simulink model "soc_dvbs2_hwtop"  (R2025b)
settings: Solver=VariableStepAuto  StartTime=0.0  StopTime=0.25  RelTol=1e-3  EnableMultiTasking=on
PreLoadFcn:
  | addpath(fullfile(matlabroot,'toolbox','whdl','whdlexamples','whdlexamples'));
InitFcn:
  | addpath(fullfile(matlabroot,'toolbox','whdl','whdlexamples','whdlexamples'));
  | soc_dvbs2_init;
values from neighbouring files (symbols this model uses):
  fs = Rsym *32    (= 128000000)    [soc_dvbs2_init.m]
  Rsym = 4e6    (= 4000000)    [soc_dvbs2_init.m]
undefined symbols (not defined in the file or in its folder): Fs, I, Q
libraries: hwlogicconnlib x2, hdlsllib x2, xilinxrfsoclib x1
CloseFcn:
  | h = warning('off','MATLAB:rmpath:DirNotFound');
  | rmpath(fullfile(matlabroot,'toolbox','whdl','whdlexamples','whdlexamples'));
  | warning(h);clear h;
settings Model: SimulationMode=accelerator  Creator=The MathWorks, Inc.  LastModifiedBy=The MathWorks, Inc.
settings SolverCC: PositivePriorityOrder=on
settings OptimizationCC: DefaultParameterBehavior=Inlined  EnhancedBackFolding=on  PassReuseOutputArgsAs=Individual arguments  ZeroExternalMemoryAtStartup=off  ZeroInternalMemoryAtStartup=off  MaxStackSize=64  OptimizeBlockOrder=speed  DifferentSizesBufferReuse=on  OptimizationCustomize=off  EfficientTunableParamExpr=on
settings DebuggingCC: ParameterTunabilityLossMsg=error
settings HardwareCC: ProdBitPerLong=64.0  ProdLargestAtomicInteger=LongLong  ProdLargestAtomicFloat=Double  ProdLongLongMode=on  ProdHWDeviceType=ARM Compatible->ARM Cortex-A (64-bit)  HardwareBoardFeatureSet=SoCBlockset
settings ModelReferenceCC: ModelReferenceNumInstancesAllowed=Single
settings SFSimCC: MATLABDynamicMemAlloc=off
settings RTWCC: SystemTargetFile=ert.tlc  HardwareBoard=Xilinx Zynq UltraScale+ RFSoC ZCU111 Evaluation Kit  TLCOptions="-aInlineSetEventsForThisBaseRateFcn=TLC_FALSE -aSuppressMultiTaskScheduler=TLC_FALSE  -aRateBasedStepFcn=0"  TemplateMakefile=ert_default_tmf  Toolchain=Linaro AArch64 Linux v6.3.1  Description=Embedded Coder
settings CodeAppCC: ForceParamTrailComments=on  IgnoreCustomStorageClasses=off  OperatorAnnotations=on  SimulinkDataObjDesc=on  SFDataObjDesc=on  InsertBlockDesc=on

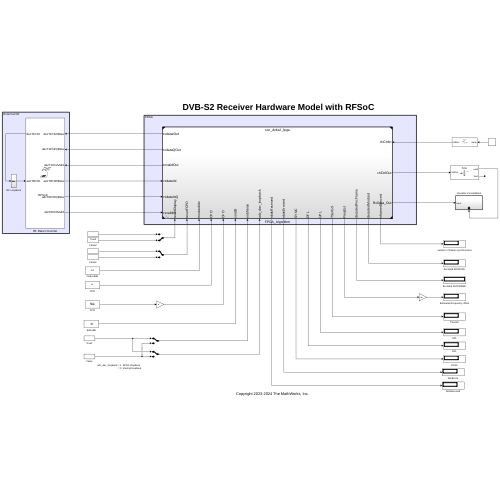
[thumbnail: Simulink's stored preview of the top-level diagram]
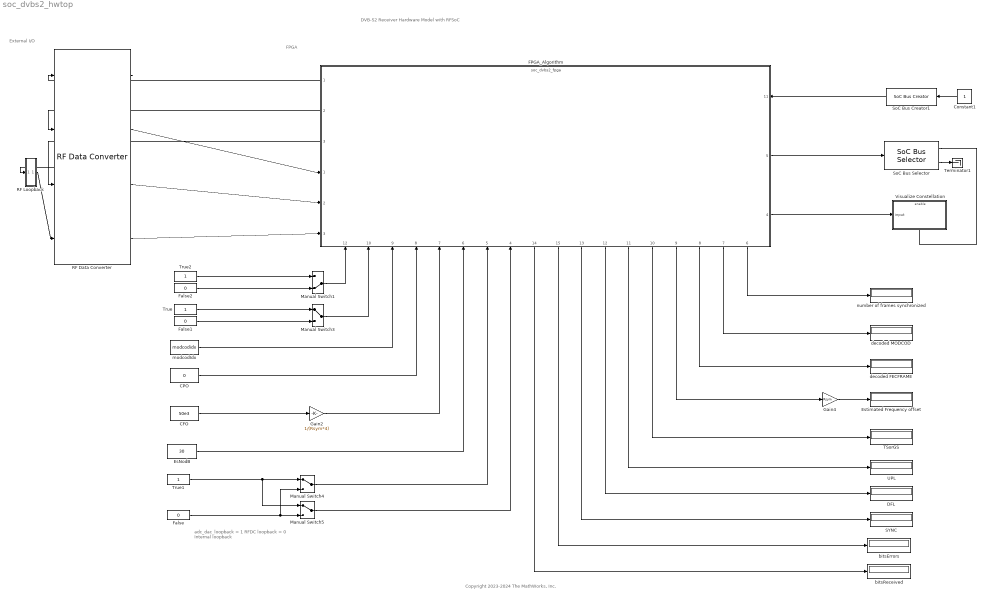
== system soc_dvbs2_hwtop ==
  note: DVB-S2 Receiver Hardware Model with RFSoC
  note: adc_dac_loopback = 1  RFDC loopback
      |                                = 0  Internal loopback
  note: External I/O
  note: FPGA
  note: Copyright 2023-2024 The MathWorks, Inc.
  CFO : Constant  Value=50e3  SampleTime=1/fs
  CPO : Constant  Value=0  OutDataTypeStr=Inherit: Inherit via back propagation  SampleTime=1/fs
  Constant1 : Constant  OutDataTypeStr=boolean  SampleTime=-1
  DFL : Display
      settings: Format=hex (Stored Integer)
  EsNodB : Constant  Value=30  OutDataTypeStr=Inherit: Inherit via back propagation  SampleTime=1/fs
  Estimated Frequency offset : Display
  FPGA_Algorithm : ModelReference  ModelNameDialog=soc_dvbs2_fpga.slx  ModelReferenceVersion=9.0
      settings: PortSchema="{\"entries\":[{\"content\":{\"sides\":[{\"content\":{\"connectorIds\":[\"Out1\",\"Out2\",\"Out3\",\"In1\",\"In2\",\"In3\"]},\"type\":\"ConnectorPlacement.EquallySpacedRectSide\",\"uuid\":\"5a98e095-40d9-43f8-91e5-a805a03516fd\"},{\"content\":{\"connectorIds\":[\"In11\",\"Out5\",\"Out4\"],\"side\":\"RIGHT\"},\"type\":\"ConnectorPlacement.EquallySpacedRectSide\",\"uuid\":\"242f1ec7-c947-482c-82ab-d4fa225331bb\"},{\"content\":{\"side\":\"TOP\"},\"type\":\"ConnectorPlacement.EquallySpacedRectSide\",\"uuid\":\"d3f55be4-91f3-4b02-af75-0bf7e7e1b925\"},{\"content\":{\"connectorIds\":[\"In12\",\"In10\",\"In9\",\"In8\",\"In7\",\"In6\",\"In5\",\"In4\",\"Out14\",\"Out15\",\"Out13\",\"Out12\",\"Out11\",\"Out10\",\"Out9\",\"Out8\",\"Out7\",\"Out6\"],\"side\":\"BOTTOM\"},\"type\":\"ConnectorPlacement.EquallySpacedRectSide\",\"uuid\":\"11ee90da-1deb-4c1f-bd41-f9aa9c63736b\"}]},\"type\":\"ConnectorPlacement.EquallySpacedConnector\",\"uuid\":\"1ac0077b-1539-4750-8893-00c30e797fc3\"}],\"packageUris\":[\"http://schema.mathworks.com/mf0/Connector/R2020b\"],\"version\":\"1.0\"}"
  False : Constant  Value=0  OutDataTypeStr=boolean  SampleTime=1/fs
  False1 : Constant  Value=0  OutDataTypeStr=boolean  SampleTime=1/fs
  False2 : Constant  Value=0  OutDataTypeStr=boolean  SampleTime=1/fs
  Gain2 : Gain  Gain=1/(Rsym*4)  OutDataTypeStr=fixdt(1,21,21)
  Gain4 : Gain  Gain=Rsym  ParamDataTypeStr=double
  Manual Switch1 : ManualSwitch  CurrentSetting=0
  Manual Switch3 : ManualSwitch
  Manual Switch4 : ManualSwitch
  Manual Switch5 : ManualSwitch
  RF Data Converter : xilinxrfsoclib/RF Data Converter  RFDCSim=Pass-through  tabPromptsCB=0  RFInterface=Customize  digitalInterface=I/Q  dac11Enable=off  dac12Enable=off  dac13Enable=off  dac14Enable=off  dac21Enable=off  dac22Enable=off  dac23Enable=on  dac24Enable=off  dac31Enable=off  dac32Enable=off  dac33Enable=off  dac34Enable=off  dac41Enable=off  dac42Enable=off  dac43Enable=off  dac44Enable=off  matchDACParam=on  dacSampleRate=2048  dacDatapathMode=Full Nyquist (0 to Fs/2)  interpolationMode=4  dacSamplesPerCycle=4  dacMixerType=Fine  dacMixerMode=I/Q->Real  dacMixerFrequency=Fs/2  dacNCOFrequency=[0.860]  dacNCOPhase=[0]  invertSyncFilter=off  dacTile1SampleRate=1000  dac11DatapathMode=Full Nyquist (0 to Fs/2)  dac11InterpolationMode=2  dac11SamplesPerCycle=2  dac11MixerType=Coarse  dac11MixerMode=I/Q->Real  dac11MixerFrequency=Fs/2  dac11NCOFrequency=0  dac11NCOPhase=0  dac11InvertSyncFilter=off  dac12DatapathMode=Full Nyquist (0 to Fs/2)  dac12InterpolationMode=2  dac12SamplesPerCycle=2  dac12MixerType=Coarse  dac12MixerMode=I/Q->Real  dac12MixerFrequency=Fs/2  dac12NCOFrequency=0  dac12NCOPhase=0  dac12InvertSyncFilter=off  dac13DatapathMode=Full Nyquist (0 to Fs/2)  dac13InterpolationMode=2  dac13SamplesPerCycle=2  dac13MixerType=Coarse  dac13MixerMode=I/Q->Real  dac13MixerFrequency=Fs/2  dac13NCOFrequency=0  dac13NCOPhase=0  dac13InvertSyncFilter=off  dac14DatapathMode=Full Nyquist (0 to Fs/2)  dac14InterpolationMode=2  dac14SamplesPerCycle=2  dac14MixerType=Coarse  dac14MixerMode=I/Q->Real  dac14MixerFrequency=Fs/2  dac14NCOFrequency=0  dac14NCOPhase=0  dac14InvertSyncFilter=off  dacTile2SampleRate=1000  dac21DatapathMode=Full Nyquist (0 to Fs/2)  dac21InterpolationMode=2  dac21SamplesPerCycle=2  dac21MixerType=Coarse  dac21MixerMode=I/Q->Real  dac21MixerFrequency=Fs/2  dac21NCOFrequency=0  dac21NCOPhase=0  dac21InvertSyncFilter=off  dac22DatapathMode=Full Nyquist (0 to Fs/2)  dac22InterpolationMode=2  dac22SamplesPerCycle=2  dac22MixerType=Coarse  dac22MixerMode=I/Q->Real  dac22MixerFrequency=Fs/2  dac22NCOFrequency=0  dac22NCOPhase=0  dac22InvertSyncFilter=off  dac23DatapathMode=Full Nyquist (0 to Fs/2)  dac23InterpolationMode=2  dac23SamplesPerCycle=2  dac23MixerType=Coarse  dac23MixerMode=I/Q->Real  dac23MixerFrequency=Fs/2  dac23NCOFrequency=0  dac23NCOPhase=0  dac23InvertSyncFilter=off  dac24DatapathMode=Full Nyquist (0 to Fs/2)  dac24InterpolationMode=2  dac24SamplesPerCycle=2  dac24MixerType=Coarse  dac24MixerMode=I/Q->Real  dac24MixerFrequency=Fs/2  dac24NCOFrequency=0  dac24NCOPhase=0  dac24InvertSyncFilter=off  dacTile3SampleRate=1000  dac31DatapathMode=Full Nyquist (0 to Fs/2)  dac31InterpolationMode=2  dac31SamplesPerCycle=2  dac31MixerType=Coarse  dac31MixerMode=I/Q->Real  dac31MixerFrequency=Fs/2  dac31NCOFrequency=0  dac31NCOPhase=0  dac31InvertSyncFilter=off  dac32DatapathMode=Full Nyquist (0 to Fs/2)  dac32InterpolationMode=2  dac32SamplesPerCycle=2  dac32MixerType=Coarse  dac32MixerMode=I/Q->Real  dac32MixerFrequency=Fs/2  dac32NCOFrequency=0  dac32NCOPhase=0  dac32InvertSyncFilter=off  dac33DatapathMode=Full Nyquist (0 to Fs/2)  dac33InterpolationMode=2  dac33SamplesPerCycle=2  dac33MixerType=Coarse  dac33MixerMode=I/Q->Real  dac33MixerFrequency=Fs/2  dac33NCOFrequency=0  dac33NCOPhase=0  dac33InvertSyncFilter=off  dac34DatapathMode=Full Nyquist (0 to Fs/2)  dac34InterpolationMode=2  dac34SamplesPerCycle=2  dac34MixerType=Coarse  dac34MixerMode=I/Q->Real  dac34MixerFrequency=Fs/2  dac34NCOFrequency=0  dac34NCOPhase=0  dac34InvertSyncFilter=off  dacTile4SampleRate=1000  dac41DatapathMode=Full Nyquist (0 to Fs/2)  dac41InterpolationMode=2  dac41SamplesPerCycle=2  dac41MixerType=Coarse  dac41MixerMode=I/Q->Real  dac41MixerFrequency=Fs/2  dac41NCOFrequency=0  dac41NCOPhase=0  dac41InvertSyncFilter=off  dac42DatapathMode=Full Nyquist (0 to Fs/2)  dac42InterpolationMode=2  dac42SamplesPerCycle=2  dac42MixerType=Coarse  dac42MixerMode=I/Q->Real  dac42MixerFrequency=Fs/2  dac42NCOFrequency=0  dac42NCOPhase=0  dac42InvertSyncFilter=off  dac43DatapathMode=Full Nyquist (0 to Fs/2)  dac43InterpolationMode=2  dac43SamplesPerCycle=2  dac43MixerType=Coarse  dac43MixerMode=I/Q->Real  dac43MixerFrequency=Fs/2  dac43NCOFrequency=0  dac43NCOPhase=0  dac43InvertSyncFilter=off  dac44DatapathMode=Full Nyquist (0 to Fs/2)  dac44InterpolationMode=2  dac44SamplesPerCycle=2  dac44MixerType=Coarse  dac44MixerMode=I/Q->Real  dac44MixerFrequency=Fs/2  dac44NCOFrequency=0  dac44NCOPhase=0  dac44InvertSyncFilter=off  adc11Enable=on  adc12Enable=off  adc13Enable=off  adc14Enable=off  adc21Enable=off  adc22Enable=off  adc23Enable=off  adc24Enable=off  adc31Enable=off  adc32Enable=off  adc33Enable=off  adc34Enable=off  adc41Enable=off  adc42Enable=off  adc43Enable=off  adc44Enable=off  adcOutUnpackedData=on  matchADCParam=on  adcSampleRate=2048  decimationMode=4  adcSamplesPerCycle=4  adcMixerType=Fine  adcMixerMode=Real->I/Q  adcMixerFrequency=Fs/2  adcNCOFrequency=[-0.860]  adcNCOPhase=[0]  adcTile1SampleRate=1000  adc11DecimationMode=2  adc11SamplesPerCycle=2  adc11MixerType=Coarse  adc11MixerMode=Real->I/Q  adc11MixerFrequency=Fs/2  adc11NCOFrequency=0  adc11NCOPhase=0  adc12DecimationMode=2  adc12SamplesPerCycle=2  adc12MixerType=Coarse  adc12MixerMode=Real->I/Q  adc12MixerFrequency=Fs/2  adc12NCOFrequency=0  adc12NCOPhase=0  adc13DecimationMode=2  adc13SamplesPerCycle=2  adc13MixerType=Coarse  adc13MixerMode=Real->I/Q  adc13MixerFrequency=Fs/2  adc13NCOFrequency=0  adc13NCOPhase=0  adc14DecimationMode=2  adc14SamplesPerCycle=2  adc14MixerType=Coarse  adc14MixerMode=Real->I/Q  adc14MixerFrequency=Fs/2  adc14NCOFrequency=0  adc14NCOPhase=0  adcTile2SampleRate=1000  adc21DecimationMode=2  adc21SamplesPerCycle=2  adc21MixerType=Coarse  adc21MixerMode=Real->I/Q  adc21MixerFrequency=Fs/2  adc21NCOFrequency=0  adc21NCOPhase=0  adc22DecimationMode=2  adc22SamplesPerCycle=2  adc22MixerType=Coarse  adc22MixerMode=Real->I/Q  adc22MixerFrequency=Fs/2  adc22NCOFrequency=0  adc22NCOPhase=0  adc23DecimationMode=2  adc23SamplesPerCycle=2  adc23MixerType=Coarse  adc23MixerMode=Real->I/Q  adc23MixerFrequency=Fs/2  adc23NCOFrequency=0  adc23NCOPhase=0  adc24DecimationMode=2  adc24SamplesPerCycle=2  adc24MixerType=Coarse  adc24MixerMode=Real->I/Q  adc24MixerFrequency=Fs/2  adc24NCOFrequency=0  adc24NCOPhase=0  adcTile3SampleRate=1000  adc31DecimationMode=2  adc31SamplesPerCycle=2  adc31MixerType=Coarse  adc31MixerMode=Real->I/Q  adc31MixerFrequency=Fs/2  adc31NCOFrequency=0  adc31NCOPhase=0  adc32DecimationMode=2  adc32SamplesPerCycle=2  adc32MixerType=Coarse  adc32MixerMode=Real->I/Q  adc32MixerFrequency=Fs/2  adc32NCOFrequency=0  adc32NCOPhase=0  adc33DecimationMode=2  adc33SamplesPerCycle=2  adc33MixerType=Coarse  adc33MixerMode=Real->I/Q  adc33MixerFrequency=Fs/2  adc33NCOFrequency=0  adc33NCOPhase=0  adc34DecimationMode=2  adc34SamplesPerCycle=2  adc34MixerType=Coarse  adc34MixerMode=Real->I/Q  adc34MixerFrequency=Fs/2  adc34NCOFrequency=0  adc34NCOPhase=0  adcTile4SampleRate=1000  adc41DecimationMode=2  adc41SamplesPerCycle=2  adc41MixerType=Coarse  adc41MixerMode=Real->I/Q  adc41MixerFrequency=Fs/2  adc41NCOFrequency=0  adc41NCOPhase=0  adc42DecimationMode=2  adc42SamplesPerCycle=2  adc42MixerType=Coarse  adc42MixerMode=Real->I/Q  adc42MixerFrequency=Fs/2  adc42NCOFrequency=0  adc42NCOPhase=0  adc43DecimationMode=2  adc43SamplesPerCycle=2  adc43MixerType=Coarse  adc43MixerMode=Real->I/Q  adc43MixerFrequency=Fs/2  adc43NCOFrequency=0  adc43NCOPhase=0  adc44DecimationMode=2  adc44SamplesPerCycle=2  adc44MixerType=Coarse  adc44MixerMode=Real->I/Q  adc44MixerFrequency=Fs/2  adc44NCOFrequency=0  adc44NCOPhase=0  multiTileSync=off  externalPLL=off  dacRealTimeNCOPortsEnable=off  adcRealTimeNCOPortsEnable=off  adcRealTimePortsEnable=off  adcThresholdMode=Sticky over  adcThreshold1=0  adcDelayCounter=0  adcThreshold2Mode=Sticky over  adcThreshold2=0  adcThreshold2DelayCounter=0  adc11ThresholdMode=Sticky over  adc11Threshold1=0  adc11DelayCounter=0  adc11Threshold2Mode=Sticky over  adc11Threshold2=0  adc11Threshold2DelayCounter=0  adc12ThresholdMode=Sticky over  adc12Threshold1=0  adc12DelayCounter=0  adc12Threshold2Mode=Sticky over  adc12Threshold2=0  adc12Threshold2DelayCounter=0  adc13ThresholdMode=Sticky over  adc13Threshold1=0  adc13DelayCounter=0  adc13Threshold2Mode=Sticky over  adc13Threshold2=0  adc13Threshold2DelayCounter=0  adc14ThresholdMode=Sticky over  adc14Threshold1=0  adc14DelayCounter=0  adc14Threshold2Mode=Sticky over  adc14Threshold2=0  adc14Threshold2DelayCounter=0  adc21ThresholdMode=Sticky over  adc21Threshold1=0  adc21DelayCounter=0  adc21Threshold2Mode=Sticky over  adc21Threshold2=0  adc21Threshold2DelayCounter=0  adc22ThresholdMode=Sticky over  adc22Threshold1=0  adc22DelayCounter=0  adc22Threshold2Mode=Sticky over  adc22Threshold2=0  adc22Threshold2DelayCounter=0  adc23ThresholdMode=Sticky over  adc23Threshold1=0  adc23DelayCounter=0  adc23Threshold2Mode=Sticky over  adc23Threshold2=0  adc23Threshold2DelayCounter=0  adc24ThresholdMode=Sticky over  adc24Threshold1=0  adc24DelayCounter=0  adc24Threshold2Mode=Sticky over  adc24Threshold2=0  adc24Threshold2DelayCounter=0  adc31ThresholdMode=Sticky over  adc31Threshold1=0  adc31DelayCounter=0  adc31Threshold2Mode=Sticky over  adc31Threshold2=0  adc31Threshold2DelayCounter=0  adc32ThresholdMode=Sticky over  adc32Threshold1=0  adc32DelayCounter=0  adc32Threshold2Mode=Sticky over  adc32Threshold2=0  adc32Threshold2DelayCounter=0  adc33ThresholdMode=Sticky over  adc33Threshold1=0  adc33DelayCounter=0  adc33Threshold2Mode=Sticky over  adc33Threshold2=0  adc33Threshold2DelayCounter=0  adc34ThresholdMode=Sticky over  adc34Threshold1=0  adc34DelayCounter=0  adc34Threshold2Mode=Sticky over  adc34Threshold2=0  adc34Threshold2DelayCounter=0  adc41ThresholdMode=Sticky over  adc41Threshold1=0  adc41DelayCounter=0  adc41Threshold2Mode=Sticky over  adc41Threshold2=0  adc41Threshold2DelayCounter=0  adc42ThresholdMode=Sticky over  adc42Threshold1=0  adc42DelayCounter=0  adc42Threshold2Mode=Sticky over  adc42Threshold2=0  adc42Threshold2DelayCounter=0  adc43ThresholdMode=Sticky over  adc43Threshold1=0  adc43DelayCounter=0  adc43Threshold2Mode=Sticky over  adc43Threshold2=0  adc43Threshold2DelayCounter=0  adc44ThresholdMode=Sticky over  adc44Threshold1=0  adc44DelayCounter=0  adc44Threshold2Mode=Sticky over  adc44Threshold2=0  adc44Threshold2DelayCounter=0
  RF Loopback : Subsystem
  SYNC : Display
  SoC Bus Creator1 : hwlogicconnlib/SoC Bus Creator  Protocol=Data stream  ctrltype=Ready
  SoC Bus Selector : hwlogicconnlib/SoC Bus Selector  Protocol=Data stream  ctrltype=Valid
  TSorGS : Display
  Terminator1 : Terminator
  True : Constant  OutDataTypeStr=boolean  SampleTime=1/fs
  True1 : Constant  OutDataTypeStr=boolean  SampleTime=1/fs
  True2 : Constant  OutDataTypeStr=boolean  SampleTime=1/fs
  UPL : Display
  Visualize Constellation : Subsystem
  bitsErrors : Display
      settings: Format=decimal (Stored Integer)
  bitsReceived : Display
      settings: Format=decimal (Stored Integer)
  decoded FECFRAME : Display
  decoded MODCOD : Display
  modcodIdx : Constant  Value=modcodidx  OutDataTypeStr=fixdt(0,5,0)  SampleTime=1/fs  mask{modcodvalue=14}
      mask prompts: modcodvalue "MODCOD :"
      mask init:
      | modcodidx = modcodvalue - 1;
      mask TypeOptions modcodvalue: 1 | 2 | 3 | 4 | 5 | 6 | 7 | 8 | 9 | 10 | 12 | 13 | 14 | 15 | 16 | 18 | 19 | 20 | 21 | 22 | 24 | 25 | 26 | 27
      mask Display: disp(get_param(gcb,'modcodvalue'));
  number of frames synchronized : Display
  wires:
  Gain2/1 -> FPGA_Algorithm/7
  True/1 -> Manual Switch3/1
  RF Loopback/1(adc) -> RF Data Converter/4
  False/1 -> Manual Switch4/2, Manual Switch5/2
  FPGA_Algorithm/1 -> RF Data Converter/1
  Manual Switch1/1 -> FPGA_Algorithm/12
  Manual Switch3/1 -> FPGA_Algorithm/10
  RF Data Converter/2 -> FPGA_Algorithm/1
  False1/1 -> Manual Switch3/2
  Manual Switch4/1 -> FPGA_Algorithm/5
  RF Data Converter/4 -> FPGA_Algorithm/3
  FPGA_Algorithm/7 -> decoded MODCOD/1
  False2/1 -> Manual Switch1/2
  SoC Bus Selector/2 -> Terminator1/1
  CFO/1 -> Gain2/1
  SoC Bus Selector/1 -> Visualize Constellation/Enable
  True1/1 -> Manual Switch5/1, Manual Switch4/1
  Constant1/1 -> SoC Bus Creator1/1
  True2/1 -> Manual Switch1/1
  FPGA_Algorithm/6 -> number of frames synchronized/1
  Manual Switch5/1 -> FPGA_Algorithm/4
  FPGA_Algorithm/8 -> decoded FECFRAME/1
  FPGA_Algorithm/5 -> SoC Bus Selector/1
  SoC Bus Creator1/1 -> FPGA_Algorithm/11
  RF Data Converter/3 -> FPGA_Algorithm/2
  EsNodB/1 -> FPGA_Algorithm/6
  CPO/1 -> FPGA_Algorithm/8
  FPGA_Algorithm/2 -> RF Data Converter/2
  RF Data Converter/1 -> RF Loopback/1(dac)
  FPGA_Algorithm/4 -> Visualize Constellation/1(input)
  FPGA_Algorithm/3 -> RF Data Converter/3
  modcodIdx/1 -> FPGA_Algorithm/9
  FPGA_Algorithm/9 -> Gain4/1
  Gain4/1 -> Estimated Frequency offset/1
  FPGA_Algorithm/10 -> TSorGS/1
  FPGA_Algorithm/11 -> UPL/1
  FPGA_Algorithm/12 -> DFL/1
  FPGA_Algorithm/13 -> SYNC/1
  FPGA_Algorithm/15 -> bitsErrors/1
  FPGA_Algorithm/14 -> bitsReceived/1

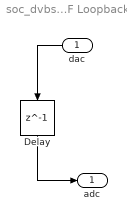
== system soc_dvbs2_hwtop/RF Loopback ==
  dac : Inport
  Delay : Delay  DelayLength=1
  adc : Outport
  wires:
  dac/1 -> Delay/1
  Delay/1 -> adc/1

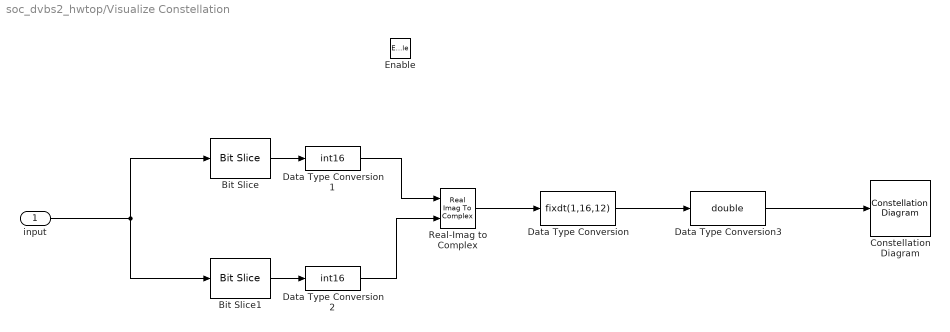
== system soc_dvbs2_hwtop/Visualize Constellation ==
  input : Inport
  Enable : EnablePort
  Bit Slice : hdlsllib/Logic and Bit Operations/Bit Slice  lidx=31  ridx=16
  Bit Slice1 : hdlsllib/Logic and Bit Operations/Bit Slice  lidx=15  ridx=0
  Constellation Diagram : ConstellationDiagram  WindowPosition=[550.000000,162.000000,254.000000,402.000000,]  Visible=on  ScopeFrameLocation=window  SymbolsToDisplaySource=Property  SymbolsToDisplay=1000  XLimits=[-1.97,1.97]  YLimits=[-1.97,1.97]  AxesLimits=[-1.97,1.97]  DefaultConfigurationName=comm.scopes.ConstellationDiagramBlockCfg
  Data Type Conversion : DataTypeConversion  OutDataTypeStr=fixdt(1,16,12)  ConvertRealWorld=Stored Integer (SI)  SaturateOnIntegerOverflow=off  RndMeth=Floor
  Data Type Conversion1 : DataTypeConversion  OutDataTypeStr=int16  ConvertRealWorld=Stored Integer (SI)  SaturateOnIntegerOverflow=off  RndMeth=Floor
  Data Type Conversion2 : DataTypeConversion  OutDataTypeStr=int16  ConvertRealWorld=Stored Integer (SI)  SaturateOnIntegerOverflow=off  RndMeth=Floor
  Data Type Conversion3 : DataTypeConversion  OutDataTypeStr=double  SaturateOnIntegerOverflow=off  RndMeth=Floor
  Real-Imag to Complex : RealImagToComplex
  wires:
  Data Type Conversion/1 -> Data Type Conversion3/1
  Data Type Conversion1/1 -> Real-Imag to Complex/1
  Bit Slice/1 -> Data Type Conversion1/1
  Bit Slice1/1 -> Data Type Conversion2/1
  Data Type Conversion2/1 -> Real-Imag to Complex/2
  input/1 -> Bit Slice1/1, Bit Slice/1
  Real-Imag to Complex/1 -> Data Type Conversion/1
  Data Type Conversion3/1 -> Constellation Diagram/1
